simulink model "AGS_controller_sim"  (R2021a)
settings: Solver=VariableStepAuto  StartTime=0.0  StopTime=inf  RelTol=1e-3
values from neighbouring files (symbols this model uses):
  Ai =     [test_matio.mat]
  Bi =     [test_matio.mat]
  Ci =     [test_matio.mat]
undefined symbols (not defined in the file or in its folder): Aki, Bki, Cki, Dki, Xi, Yi
libraries: simulink x3
settings Model: Creator=bascetta  LastModifiedBy=bascetta
settings DataIOCC: FinalStateName=PID_controller_simSimState  SaveFinalState=on  SaveOperatingPoint=on  SaveOutput=off  SignalLogging=off  DSMLogging=off  SaveTime=off  ReturnWorkspaceOutputs=off

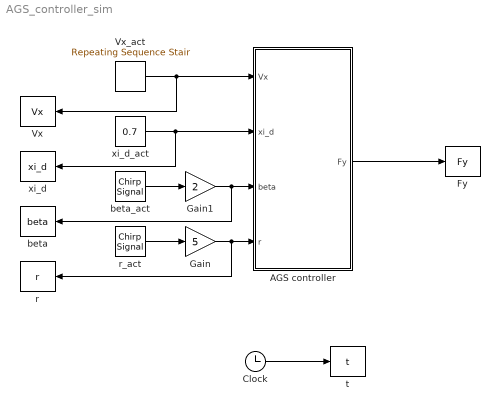
== system AGS_controller_sim ==
  AGS controller : Subsystem  mask{Ak0=Aki{1}, Ak1=Aki{2}, Ak2=Aki{3}, Ak3=Aki{4}, Bk0=Bki{1}, Bk1=Bki{2}, Bk2=Bki{3}, Bk3=Bki{4}, Ck0=Cki{1}, Ck1=Cki{2}, Ck2=Cki{3}, Ck3=Cki{4}, Dk0=Dki{1}, Dk1=Dki{2}, Dk2=Dki{3}, Dk3=Dki{4}, A0=Ai{1}, A1=Ai{2}, A2=Ai{3}, A3=Ai{4}, B0=Bi{1}, B1=Bi{2}, B2=Bi{3}, B3=Bi{4}, C0=Ci{1}, C1=Ci{2}, C2=Ci{3}, C3=Ci{4}, X0=Xi{1}, Y0=Yi{1}, Y1=Yi{2}, Y2=Yi{3}, Y3=Yi{4}}
      mask DialogControl Container3 Prompt: Controller
      mask DialogControl Container4 Prompt: Plant
      mask DialogControl Container5 Prompt: Lyapunov
  Clock : Clock
  Fy : ToWorkspace  VariableName=Fy  SampleTime=0.010000
      settings: Save2DSignal=2-D array (concatenate along first dimension)
  Gain : Gain  Gain=5
  Gain1 : Gain  Gain=2
  Vx : ToWorkspace  VariableName=Vx  SampleTime=0.010000
      settings: Save2DSignal=2-D array (concatenate along first dimension)
  Vx_act : simulink/Sources/Repeating Sequence Stair  OutValues=[5:2:15].'  tsamp=5  OutMin=[]  OutMax=[]  OutDataTypeStr=double  OutputDataTypeScalingMode=double  OutDataType=fixdt(0,8)  ConRadixGroup=Best Precision: Vector-wise  OutScaling=2^-12
  beta : ToWorkspace  VariableName=beta  SampleTime=0.010000
      settings: Save2DSignal=2-D array (concatenate along first dimension)
  beta_act : simulink/Sources/Chirp Signal  f1=0.1  T=20  f2=10
  r : ToWorkspace  VariableName=r  SampleTime=0.010000
      settings: Save2DSignal=2-D array (concatenate along first dimension)
  r_act : simulink/Sources/Chirp Signal  f1=0.1  T=20  f2=10
  t : ToWorkspace  VariableName=t  SampleTime=0.010000
      settings: Save2DSignal=2-D array (concatenate along first dimension)
  xi_d : ToWorkspace  VariableName=xi_d  SampleTime=0.010000
      settings: Save2DSignal=2-D array (concatenate along first dimension)
  xi_d_act : Constant  Value=0.7
  wires:
  Clock/1 -> t/1
  Vx_act/1 -> Vx/1, AGS controller/1(Vx)
  xi_d_act/1 -> xi_d/1, AGS controller/2(xi_d)
  AGS controller/1(Fy) -> Fy/1
  r_act/1 -> Gain/1
  Gain/1 -> r/1, AGS controller/4(r)
  beta_act/1 -> Gain1/1
  Gain1/1 -> beta/1, AGS controller/3(beta)

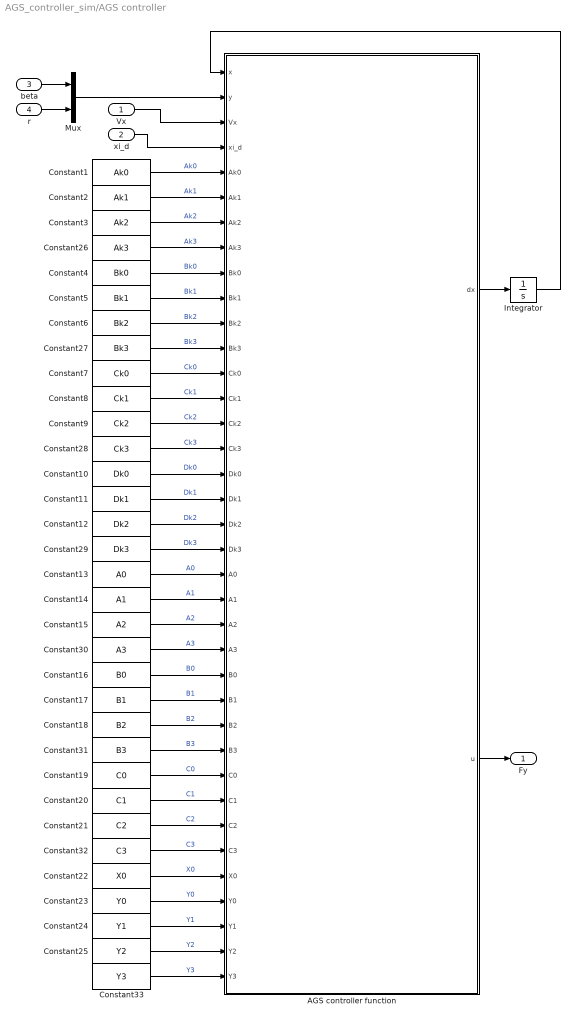
== system AGS_controller_sim/AGS controller ==
  Vx : Inport
  xi_d : Inport  Port=2
  beta : Inport  Port=3
  r : Inport  Port=4
  AGS controller function : MATLAB Function  TreatAsAtomicUnit=on
  Constant1 : Constant  Value=Ak0  VectorParams1D=off
  Constant10 : Constant  Value=Dk0  VectorParams1D=off
  Constant11 : Constant  Value=Dk1  VectorParams1D=off
  Constant12 : Constant  Value=Dk2  VectorParams1D=off
  Constant13 : Constant  Value=A0  VectorParams1D=off
  Constant14 : Constant  Value=A1  VectorParams1D=off
  Constant15 : Constant  Value=A2  VectorParams1D=off
  Constant16 : Constant  Value=B0  VectorParams1D=off
  Constant17 : Constant  Value=B1  VectorParams1D=off
  Constant18 : Constant  Value=B2  VectorParams1D=off
  Constant19 : Constant  Value=C0  VectorParams1D=off
  Constant2 : Constant  Value=Ak1  VectorParams1D=off
  Constant20 : Constant  Value=C1  VectorParams1D=off
  Constant21 : Constant  Value=C2  VectorParams1D=off
  Constant22 : Constant  Value=X0  VectorParams1D=off
  Constant23 : Constant  Value=Y0  VectorParams1D=off
  Constant24 : Constant  Value=Y1  VectorParams1D=off
  Constant25 : Constant  Value=Y2  VectorParams1D=off
  Constant26 : Constant  Value=Ak3  VectorParams1D=off
  Constant27 : Constant  Value=Bk3  VectorParams1D=off
  Constant28 : Constant  Value=Ck3  VectorParams1D=off
  Constant29 : Constant  Value=Dk3  VectorParams1D=off
  Constant3 : Constant  Value=Ak2  VectorParams1D=off
  Constant30 : Constant  Value=A3  VectorParams1D=off
  Constant31 : Constant  Value=B3  VectorParams1D=off
  Constant32 : Constant  Value=C3  VectorParams1D=off
  Constant33 : Constant  Value=Y3  VectorParams1D=off
  Constant4 : Constant  Value=Bk0  VectorParams1D=off
  Constant5 : Constant  Value=Bk1  VectorParams1D=off
  Constant6 : Constant  Value=Bk2  VectorParams1D=off
  Constant7 : Constant  Value=Ck0  VectorParams1D=off
  Constant8 : Constant  Value=Ck1  VectorParams1D=off
  Constant9 : Constant  Value=Ck2  VectorParams1D=off
  Integrator : Integrator
  Mux : Mux  Inputs=2
  Fy : Outport
  wires:
  Integrator/1 -> AGS controller function/1(x)
  Vx/1 -> AGS controller function/3(Vx)
  AGS controller function/1(dx) -> Integrator/1
  AGS controller function/2(u) -> Fy/1
  Constant2/1 -> AGS controller function/6(Ak1)  "Ak1"
  Constant3/1 -> AGS controller function/7(Ak2)  "Ak2"
  Constant4/1 -> AGS controller function/9(Bk0)  "Bk0"
  Constant5/1 -> AGS controller function/10(Bk1)  "Bk1"
  Constant6/1 -> AGS controller function/11(Bk2)  "Bk2"
  Constant7/1 -> AGS controller function/13(Ck0)  "Ck0"
  Constant8/1 -> AGS controller function/14(Ck1)  "Ck1"
  Constant9/1 -> AGS controller function/15(Ck2)  "Ck2"
  Constant10/1 -> AGS controller function/17(Dk0)  "Dk0"
  Constant11/1 -> AGS controller function/18(Dk1)  "Dk1"
  Constant12/1 -> AGS controller function/19(Dk2)  "Dk2"
  Constant13/1 -> AGS controller function/21(A0)  "A0"
  Constant14/1 -> AGS controller function/22(A1)  "A1"
  Constant15/1 -> AGS controller function/23(A2)  "A2"
  Constant18/1 -> AGS controller function/27(B2)  "B2"
  Constant16/1 -> AGS controller function/25(B0)  "B0"
  Constant17/1 -> AGS controller function/26(B1)  "B1"
  Constant19/1 -> AGS controller function/29(C0)  "C0"
  Constant20/1 -> AGS controller function/30(C1)  "C1"
  Constant21/1 -> AGS controller function/31(C2)  "C2"
  Constant22/1 -> AGS controller function/33(X0)  "X0"
  Constant23/1 -> AGS controller function/34(Y0)  "Y0"
  Constant24/1 -> AGS controller function/35(Y1)  "Y1"
  Constant25/1 -> AGS controller function/36(Y2)  "Y2"
  xi_d/1 -> AGS controller function/4(xi_d)
  Constant1/1 -> AGS controller function/5(Ak0)  "Ak0"
  Constant26/1 -> AGS controller function/8(Ak3)  "Ak3"
  Constant27/1 -> AGS controller function/12(Bk3)  "Bk3"
  Constant28/1 -> AGS controller function/16(Ck3)  "Ck3"
  Constant29/1 -> AGS controller function/20(Dk3)  "Dk3"
  Constant30/1 -> AGS controller function/24(A3)  "A3"
  Constant31/1 -> AGS controller function/28(B3)  "B3"
  Constant32/1 -> AGS controller function/32(C3)  "C3"
  Constant33/1 -> AGS controller function/37(Y3)  "Y3"
  r/1 -> Mux/2
  beta/1 -> Mux/1
  Mux/1 -> AGS controller function/2(y)

== matlab function AGS_controller_sim/AGS controller/AGS controller function ==
  data: x input; y input; dx output; Vx input; xi_d input; u output; Ak0 input; Ak1 input; Ak2 input; Ak3 input; Bk0 input; Bk1 input; Bk2 input; Bk3 input; Ck0 input; Ck1 input; Ck2 input; Ck3 input; Dk0 input; Dk1 input; Dk2 input; Dk3 input; A0 input; A1 input; A2 input; A3 input; B0 input; B1 input; B2 input; B3 input; C0 input; C1 input; C2 input; C3 input; X0 input; Y0 input; Y1 input; Y2 input; Y3 input
function [dx,u] = AGS_controller(x,y,Vx,xi_d,Ak0,Ak1,Ak2,Ak3,Bk0,Bk1,Bk2,Bk3,Ck0,Ck1,Ck2,Ck3,Dk0,Dk1,Dk2,Dk3,...
    A0,A1,A2,A3,B0,B1,B2,B3,C0,C1,C2,C3,X0,Y0,Y1,Y2,Y3)

% Compute X and Y
X = X0;
Y = Y0+Y1/Vx+Y2/Vx^2+Y3*xi_d;

% Compute hat and plant matrices
Ak_hat = Ak0+Ak1/Vx+Ak2/Vx^2+Ak3*xi_d;
Bk_hat = Bk0+Bk1/Vx+Bk2/Vx^2+Bk3*xi_d;
Ck_hat = Ck0+Ck1/Vx+Ck2/Vx^2+Ck3*xi_d;
Dk_hat = Dk0+Dk1/Vx+Dk2/Vx^2+Dk3*xi_d;

A = A0+A1/Vx+A2/Vx^2+A3*xi_d;
B = B0+B1/Vx+B2/Vx^2+B3*xi_d;
C = C0+C1/Vx+C2/Vx^2+C3*xi_d;

% Compute controller matrices
NMt = eye(size(X)) - X*Y;
[N,Mt] = lu(NMt);
M = Mt';

Ak = N\(Ak_hat-X*(A-B*Dk_hat*C)*Y-Bk_hat*C*Y-X*B*Ck_hat)/(M');
Bk = N\(Bk_hat-X*B*Dk_hat);
Ck = (Ck_hat-Dk_hat*C*Y)/(M');
Dk = Dk_hat;

% Controller equations
dx = zeros(size(Ak,1),1);
u  = zeros(1,1);

dx = Ak*x+Bk*y;
u  = Ck*x+Dk*y;
